simulink model "statefeedback"  (Simulink 5.0)
settings: Solver=ode1  StartTime=0.0  StopTime=1000  RelTol=1e-3
InitFcn:
  | init_c
undefined symbols (not defined in the file): a, dzcv, fc, fp, fs, g, j, l, mi, xc, yc
settings Model: LastModifiedBy=AD  BooleanDataType=off

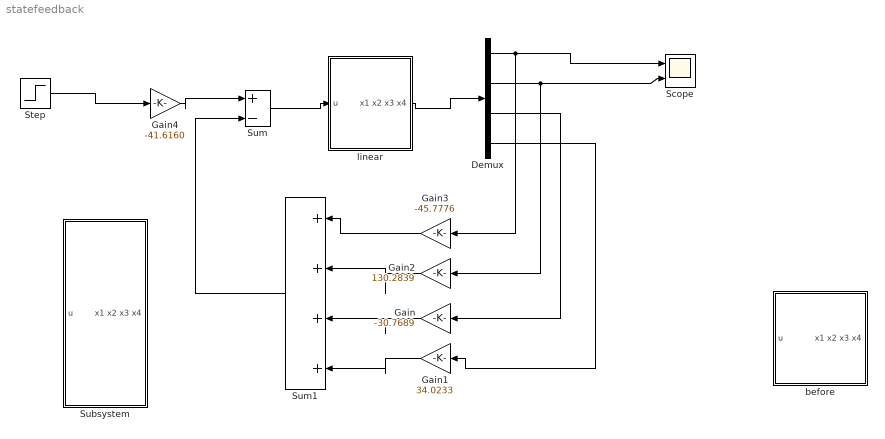
== system statefeedback ==
  Demux : Demux
  Gain : Gain  Orientation=left  Gain=-30.7689  SaturateOnIntegerOverflow=on
  Gain1 : Gain  Orientation=left  Gain=34.0233  SaturateOnIntegerOverflow=on
  Gain2 : Gain  Orientation=left  Gain=130.2839  SaturateOnIntegerOverflow=on
  Gain3 : Gain  Orientation=left  Gain=-45.7776  SaturateOnIntegerOverflow=on
  Gain4 : Gain  Gain=-41.6160  SaturateOnIntegerOverflow=on
  Scope : Scope  NumInputPorts=2
      settings: TimeRange=10  YMin=-100~0  YMax=500~120
  Step : Step  SampleTime=0
  Subsystem : Subsystem
  Sum : Sum  Inputs=|+-  SaturateOnIntegerOverflow=on
  Sum1 : Sum  Orientation=left  Inputs=|++++  SaturateOnIntegerOverflow=on
  before : Subsystem
  linear : Subsystem
  wires:
  linear/1(x1 x2 x3 x4) -> Demux/1
  Demux/1 -> Gain3/1, Scope/1
  Demux/2 -> Scope/2, Gain2/1
  Demux/3 -> Gain/1
  Demux/4 -> Gain1/1
  Gain3/1 -> Sum1/1
  Gain2/1 -> Sum1/2
  Gain/1 -> Sum1/3
  Gain1/1 -> Sum1/4
  Sum1/1 -> Sum/2
  Gain4/1 -> Sum/1
  Sum/1 -> linear/1(u)
  Step/1 -> Gain4/1

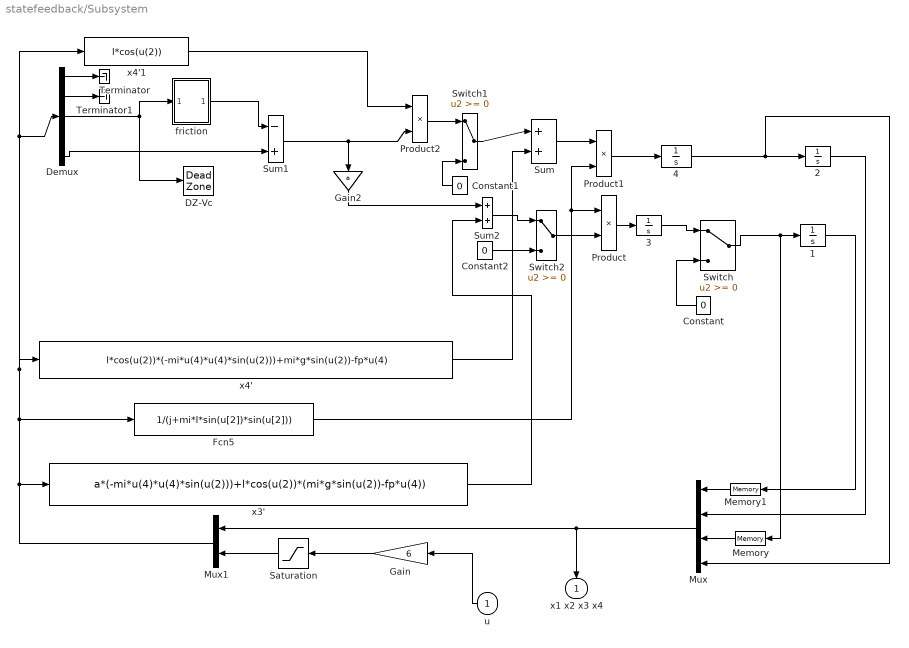
== system statefeedback/Subsystem ==
  u : Inport  Orientation=left
  {1..4} (4 alike) : Integrator
  Constant : Constant  Orientation=left  Value=0
  Constant1 : Constant  Orientation=left  Value=0
  Constant2 : Constant  Value=0
  DZ-Vc : DeadZone  LowerValue=-0.00793711  UpperValue=0.00793711  SaturateOnIntegerOverflow=on
  Demux : Demux  Outputs=5
  Fcn5 : Fcn  Expr=1/(j+mi*l*sin(u[2])*sin(u[2]))
  Gain : Gain  Orientation=left  Gain=6  SaturateOnIntegerOverflow=on
  Gain2 : Gain  Orientation=down  Gain=a  SaturateOnIntegerOverflow=on
  Memory : Memory  Orientation=left
  Memory1 : Memory  Orientation=left
  Mux : Mux  Orientation=left
  Mux1 : Mux  Orientation=left  Inputs=2
  Product : Product  SaturateOnIntegerOverflow=on
  Product1 : Product  SaturateOnIntegerOverflow=on
  Product2 : Product  SaturateOnIntegerOverflow=on
  Saturation : Saturate  Orientation=left  UpperLimit=5  LowerLimit=-5
  Sum : Sum  Inputs=|++  SaturateOnIntegerOverflow=on
  Sum1 : Sum  Inputs=-+  SaturateOnIntegerOverflow=on
  Sum2 : Sum  SaturateOnIntegerOverflow=on
  Switch : Switch  SaturateOnIntegerOverflow=on
  Switch1 : Switch  SaturateOnIntegerOverflow=on
  Switch2 : Switch  SaturateOnIntegerOverflow=on
  Terminator : Terminator
  Terminator1 : Terminator
  friction : Subsystem
  x3' : Fcn  Expr=a*(-mi*u(4)*u(4)*sin(u(2)))+l*cos(u(2))*(mi*g*sin(u(2))-fp*u(4))
  x4' : Fcn  Expr=l*cos(u(2))*(-mi*u(4)*u(4)*sin(u(2)))+mi*g*sin(u(2))-fp*u(4)
  x4'1 : Fcn  Expr=l*cos(u(2))
  x1 x2 x3 x4 : Outport  Orientation=down
  wires:
  u/1 -> Gain/1
  Demux/3 -> DZ-Vc/1, friction/1(In1)
  Constant1/1 -> Switch1/3
  Constant/1 -> Switch/3
  x4'1/1 -> Product2/1
  Product2/1 -> Switch1/1
  Switch1/1 -> Sum/1
  x4'/1 -> Sum/2
  Fcn5/1 -> Product1/2, Product/1
  Product1/1 -> 4/1
  Product/1 -> 3/1
  Gain/1 -> Saturation/1
  Mux1/1 -> x3'/1, Fcn5/1, x4'/1, x4'1/1, Demux/1
  Mux/1 -> Mux1/1, x1 x2 x3 x4/1
  Saturation/1 -> Mux1/2
  Switch/1 -> 1/1, Memory/1
  3/1 -> Switch/1
  2/1 -> Mux/2
  1/1 -> Memory1/1
  Memory/1 -> Mux/3
  Sum/1 -> Product1/1
  Switch2/1 -> Product/2
  Constant2/1 -> Switch2/3
  Memory1/1 -> Mux/1
  Sum2/1 -> Switch2/1
  x3'/1 -> Sum2/2
  Gain2/1 -> Sum2/1
  Demux/1 -> Terminator/1
  Demux/2 -> Terminator1/1
  4/1 -> 2/1, Mux/4
  Demux/5 -> Sum1/2
  Sum1/1 -> Product2/2, Gain2/1
  ? -> Switch/2, Switch1/2, Switch2/2
  friction/1(out-1) -> Sum1/1

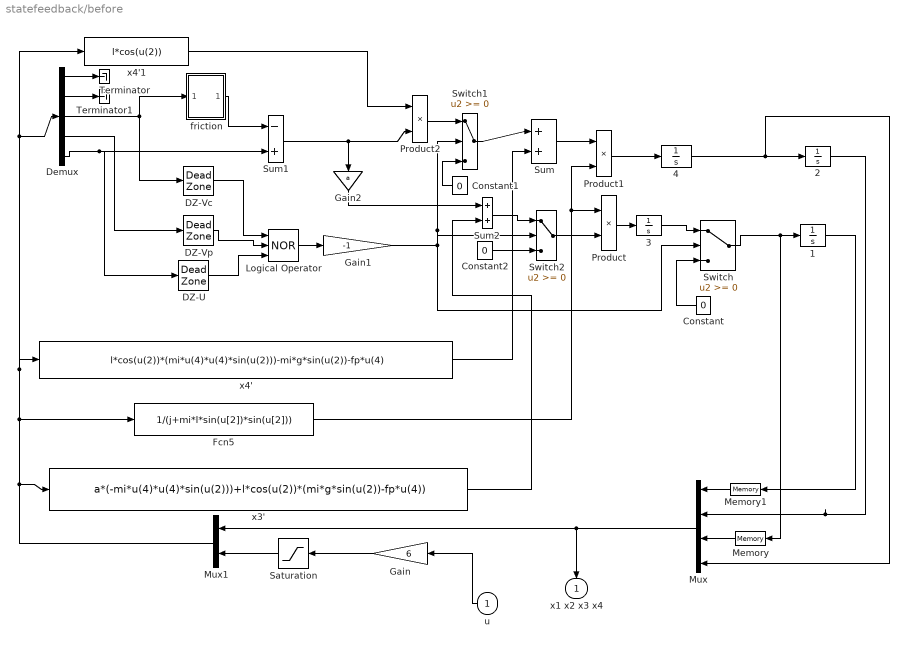
== system statefeedback/before ==
  u : Inport  Orientation=left
  {1..4} (4 alike) : Integrator
  Constant : Constant  Orientation=left  Value=0
  Constant1 : Constant  Orientation=left  Value=0
  Constant2 : Constant  Value=0
  DZ-U : DeadZone  LowerValue=-1.37918  UpperValue=1.37918  SaturateOnIntegerOverflow=on
  DZ-Vc : DeadZone  LowerValue=-0.00793711  UpperValue=0.00793711  SaturateOnIntegerOverflow=on
  DZ-Vp : DeadZone  LowerValue=-3.37476  UpperValue=3.37476  SaturateOnIntegerOverflow=on
  Demux : Demux  Outputs=5
  Fcn5 : Fcn  Expr=1/(j+mi*l*sin(u[2])*sin(u[2]))
  Gain : Gain  Orientation=left  Gain=6  SaturateOnIntegerOverflow=on
  Gain1 : Gain  Gain=-1  SaturateOnIntegerOverflow=on
  Gain2 : Gain  Orientation=down  Gain=a  SaturateOnIntegerOverflow=on
  Logical Operator : Logic  Operator=NOR  Inputs=3  AllPortsSameDT=off
  Memory : Memory  Orientation=left
  Memory1 : Memory  Orientation=left
  Mux : Mux  Orientation=left
  Mux1 : Mux  Orientation=left  Inputs=2
  Product : Product  SaturateOnIntegerOverflow=on
  Product1 : Product  SaturateOnIntegerOverflow=on
  Product2 : Product  SaturateOnIntegerOverflow=on
  Saturation : Saturate  Orientation=left  UpperLimit=5  LowerLimit=-5
  Sum : Sum  Inputs=|++  SaturateOnIntegerOverflow=on
  Sum1 : Sum  Inputs=-+  SaturateOnIntegerOverflow=on
  Sum2 : Sum  SaturateOnIntegerOverflow=on
  Switch : Switch  SaturateOnIntegerOverflow=on
  Switch1 : Switch  SaturateOnIntegerOverflow=on
  Switch2 : Switch  SaturateOnIntegerOverflow=on
  Terminator : Terminator
  Terminator1 : Terminator
  friction : Subsystem
  x3' : Fcn  Expr=a*(-mi*u(4)*u(4)*sin(u(2)))+l*cos(u(2))*(mi*g*sin(u(2))-fp*u(4))
  x4' : Fcn  Expr=l*cos(u(2))*(mi*u(4)*u(4)*sin(u(2)))-mi*g*sin(u(2))-fp*u(4)
  x4'1 : Fcn  Expr=l*cos(u(2))
  x1 x2 x3 x4 : Outport  Orientation=down
  wires:
  Gain1/1 -> Switch2/2, Switch1/2, Switch/2
  Sum1/1 -> Gain2/1, Product2/2
  Demux/5 -> Sum1/2, DZ-U/1
  4/1 -> Mux/4, 2/1
  friction/1(out-1) -> Sum1/1
  Demux/2 -> Terminator1/1
  Demux/1 -> Terminator/1
  Gain2/1 -> Sum2/1
  x3'/1 -> Sum2/2
  Sum2/1 -> Switch2/1
  Memory1/1 -> Mux/1
  Constant2/1 -> Switch2/3
  Switch2/1 -> Product/2
  Logical Operator/1 -> Gain1/1
  DZ-U/1 -> Logical Operator/3
  DZ-Vp/1 -> Logical Operator/2
  DZ-Vc/1 -> Logical Operator/1
  Sum/1 -> Product1/1
  Memory/1 -> Mux/3
  1/1 -> Memory1/1
  2/1 -> Mux/2
  3/1 -> Switch/1
  Switch/1 -> Memory/1, 1/1
  Saturation/1 -> Mux1/2
  Mux/1 -> x1 x2 x3 x4/1, Mux1/1
  Mux1/1 -> Demux/1, x4'1/1, x4'/1, Fcn5/1, x3'/1
  Gain/1 -> Saturation/1
  Product/1 -> 3/1
  Product1/1 -> 4/1
  Fcn5/1 -> Product/1, Product1/2
  x4'/1 -> Sum/2
  Switch1/1 -> Sum/1
  Product2/1 -> Switch1/1
  x4'1/1 -> Product2/1
  Constant/1 -> Switch/3
  Constant1/1 -> Switch1/3
  Demux/4 -> DZ-Vp/1
  Demux/3 -> DZ-Vc/1, friction/1(In1)
  u/1 -> Gain/1

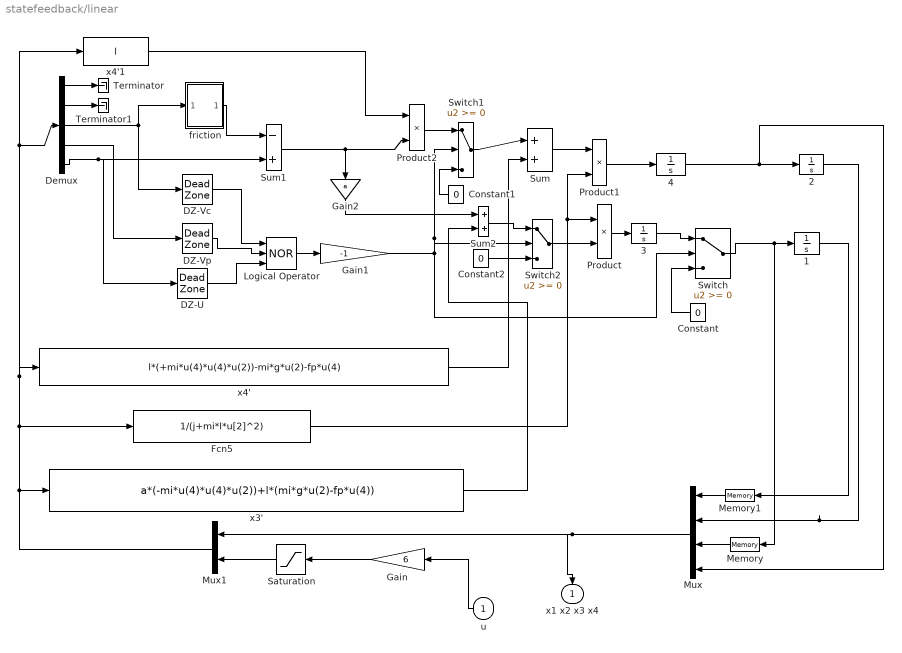
== system statefeedback/linear ==
  u : Inport  Orientation=left
  {1..4} (4 alike) : Integrator
  Constant : Constant  Orientation=left  Value=0
  Constant1 : Constant  Orientation=left  Value=0
  Constant2 : Constant  Value=0
  DZ-U : DeadZone  LowerValue=-1.37918  UpperValue=1.37918  SaturateOnIntegerOverflow=on
  DZ-Vc : DeadZone  LowerValue=-0.00793711  UpperValue=0.00793711  SaturateOnIntegerOverflow=on
  DZ-Vp : DeadZone  LowerValue=-3.37476  UpperValue=3.37476  SaturateOnIntegerOverflow=on
  Demux : Demux  Outputs=5
  Fcn5 : Fcn  Expr=1/(j+mi*l*u[2]^2)
  Gain : Gain  Orientation=left  Gain=6  SaturateOnIntegerOverflow=on
  Gain1 : Gain  Gain=-1  SaturateOnIntegerOverflow=on
  Gain2 : Gain  Orientation=down  Gain=a  SaturateOnIntegerOverflow=on
  Logical Operator : Logic  Operator=NOR  Inputs=3  AllPortsSameDT=off
  Memory : Memory  Orientation=left
  Memory1 : Memory  Orientation=left
  Mux : Mux  Orientation=left
  Mux1 : Mux  Orientation=left  Inputs=2
  Product : Product  SaturateOnIntegerOverflow=on
  Product1 : Product  SaturateOnIntegerOverflow=on
  Product2 : Product  SaturateOnIntegerOverflow=on
  Saturation : Saturate  Orientation=left  UpperLimit=5  LowerLimit=-5
  Sum : Sum  Inputs=|++  SaturateOnIntegerOverflow=on
  Sum1 : Sum  Inputs=-+  SaturateOnIntegerOverflow=on
  Sum2 : Sum  SaturateOnIntegerOverflow=on
  Switch : Switch  SaturateOnIntegerOverflow=on
  Switch1 : Switch  SaturateOnIntegerOverflow=on
  Switch2 : Switch  SaturateOnIntegerOverflow=on
  Terminator : Terminator
  Terminator1 : Terminator
  friction : Subsystem
  x3' : Fcn  Expr=a*(-mi*u(4)*u(4)*u(2))+l*(mi*g*u(2)-fp*u(4))
  x4' : Fcn  Expr=l*(+mi*u(4)*u(4)*u(2))-mi*g*u(2)-fp*u(4)
  x4'1 : Fcn  Expr=l
  x1 x2 x3 x4 : Outport  Orientation=down
  wires:
  u/1 -> Gain/1
  Demux/3 -> friction/1(In1), DZ-Vc/1
  Demux/4 -> DZ-Vp/1
  Constant1/1 -> Switch1/3
  Constant/1 -> Switch/3
  x4'1/1 -> Product2/1
  Product2/1 -> Switch1/1
  Switch1/1 -> Sum/1
  x4'/1 -> Sum/2
  Fcn5/1 -> Product1/2, Product/1
  Product1/1 -> 4/1
  Product/1 -> 3/1
  Gain/1 -> Saturation/1
  Mux1/1 -> x3'/1, Fcn5/1, x4'/1, x4'1/1, Demux/1
  Mux/1 -> Mux1/1, x1 x2 x3 x4/1
  Saturation/1 -> Mux1/2
  Switch/1 -> 1/1, Memory/1
  3/1 -> Switch/1
  2/1 -> Mux/2
  1/1 -> Memory1/1
  Memory/1 -> Mux/3
  Sum/1 -> Product1/1
  DZ-Vc/1 -> Logical Operator/1
  DZ-Vp/1 -> Logical Operator/2
  DZ-U/1 -> Logical Operator/3
  Logical Operator/1 -> Gain1/1
  Switch2/1 -> Product/2
  Constant2/1 -> Switch2/3
  Memory1/1 -> Mux/1
  Sum2/1 -> Switch2/1
  x3'/1 -> Sum2/2
  Gain2/1 -> Sum2/1
  Demux/1 -> Terminator/1
  Demux/2 -> Terminator1/1
  friction/1(out-1) -> Sum1/1
  4/1 -> 2/1, Mux/4
  Demux/5 -> DZ-U/1, Sum1/2
  Sum1/1 -> Product2/2, Gain2/1
  Gain1/1 -> Switch/2, Switch1/2, Switch2/2

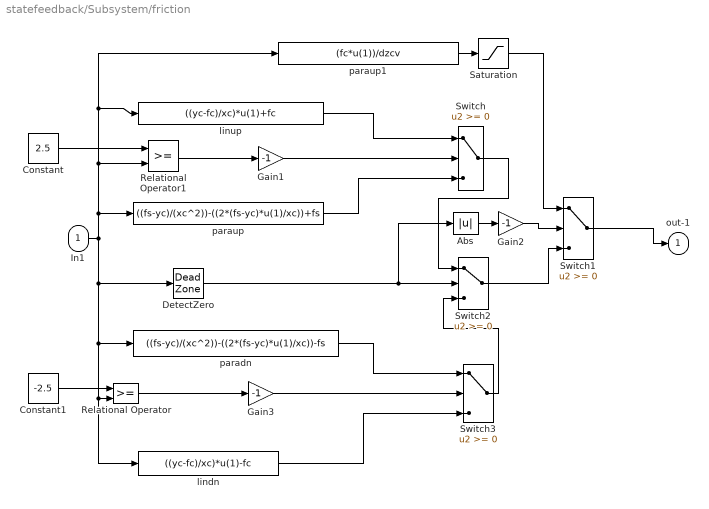
== system statefeedback/Subsystem/friction ==
  In1 : Inport
  Abs : Abs  SaturateOnIntegerOverflow=on
  Constant : Constant  Value=2.5
  Constant1 : Constant  Value=-2.5
  DetectZero : DeadZone  SaturateOnIntegerOverflow=on
  Gain1 : Gain  Gain=-1  SaturateOnIntegerOverflow=on
  Gain2 : Gain  Gain=-1  SaturateOnIntegerOverflow=on
  Gain3 : Gain  Gain=-1  SaturateOnIntegerOverflow=on
  Relational Operator : RelationalOperator
  Relational Operator1 : RelationalOperator
  Saturation : Saturate
  Switch{,1..3} (4 alike) : Switch  SaturateOnIntegerOverflow=on
  lindn : Fcn  Expr=((yc-fc)/xc)*u(1)-fc
  linup : Fcn  Expr=((yc-fc)/xc)*u(1)+fc
  paradn : Fcn  Expr=((fs-yc)/(xc^2))-((2*(fs-yc)*u(1)/xc))-fs
  paraup : Fcn  Expr=((fs-yc)/(xc^2))-((2*(fs-yc)*u(1)/xc))+fs
  paraup1 : Fcn  Expr=(fc*u(1))/dzcv
  out-1 : Outport
  wires:
  Switch1/1 -> out-1/1
  Saturation/1 -> Switch1/1
  linup/1 -> Switch/1
  paraup/1 -> Switch/3
  In1/1 -> paradn/1, Relational Operator/2, lindn/1, DetectZero/1, paraup/1, Relational Operator1/2, linup/1, paraup1/1
  DetectZero/1 -> Switch2/2, Abs/1
  Switch/1 -> Switch2/1
  Abs/1 -> Gain2/1
  Gain2/1 -> Switch1/2
  Switch2/1 -> Switch1/3
  Switch3/1 -> Switch2/3
  paradn/1 -> Switch3/1
  Relational Operator/1 -> Gain3/1
  lindn/1 -> Switch3/3
  Constant/1 -> Relational Operator1/1
  Constant1/1 -> Relational Operator/1
  Relational Operator1/1 -> Gain1/1
  paraup1/1 -> Saturation/1
  Gain1/1 -> Switch/2
  Gain3/1 -> Switch3/2

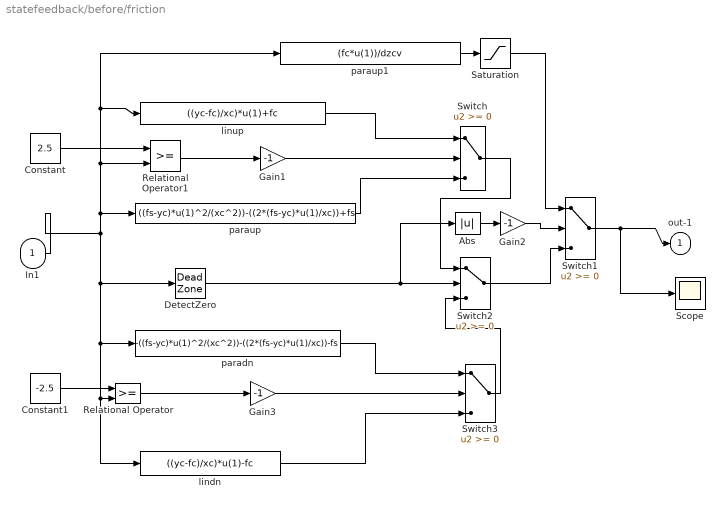
== system statefeedback/before/friction ==
  In1 : Inport
  Abs : Abs  SaturateOnIntegerOverflow=on
  Constant : Constant  Value=2.5
  Constant1 : Constant  Value=-2.5
  DetectZero : DeadZone  LowerValue=0  UpperValue=0  SaturateOnIntegerOverflow=on
  Gain1 : Gain  Gain=-1  SaturateOnIntegerOverflow=on
  Gain2 : Gain  Gain=-1  SaturateOnIntegerOverflow=on
  Gain3 : Gain  Gain=-1  SaturateOnIntegerOverflow=on
  Relational Operator : RelationalOperator
  Relational Operator1 : RelationalOperator
  Saturation : Saturate  UpperLimit=fs  LowerLimit=-fs
  Scope : Scope
      settings: SaveName=ScopeData2
  Switch{,1..3} (4 alike) : Switch  SaturateOnIntegerOverflow=on
  lindn : Fcn  Expr=((yc-fc)/xc)*u(1)-fc
  linup : Fcn  Expr=((yc-fc)/xc)*u(1)+fc
  paradn : Fcn  Expr=-((fs-yc)*u(1)^2/(xc^2))-((2*(fs-yc)*u(1)/xc))-fs
  paraup : Fcn  Expr=((fs-yc)*u(1)^2/(xc^2))-((2*(fs-yc)*u(1)/xc))+fs
  paraup1 : Fcn  Expr=(fc*u(1))/dzcv
  out-1 : Outport
  wires:
  Gain3/1 -> Switch3/2
  Gain1/1 -> Switch/2
  paraup1/1 -> Saturation/1
  Relational Operator1/1 -> Gain1/1
  Constant1/1 -> Relational Operator/1
  Constant/1 -> Relational Operator1/1
  lindn/1 -> Switch3/3
  Relational Operator/1 -> Gain3/1
  paradn/1 -> Switch3/1
  Switch3/1 -> Switch2/3
  Switch2/1 -> Switch1/3
  Gain2/1 -> Switch1/2
  Abs/1 -> Gain2/1
  Switch/1 -> Switch2/1
  DetectZero/1 -> Abs/1, Switch2/2
  paraup/1 -> Switch/3
  linup/1 -> Switch/1
  Saturation/1 -> Switch1/1
  Switch1/1 -> out-1/1, Scope/1
  In1/1 -> paraup1/1, linup/1, Relational Operator1/2, paraup/1, DetectZero/1, lindn/1, Relational Operator/2, paradn/1

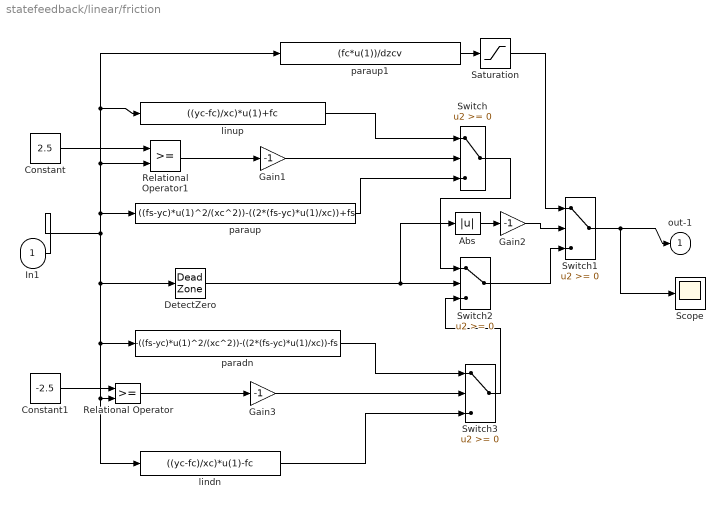
== system statefeedback/linear/friction ==
  In1 : Inport
  Abs : Abs  SaturateOnIntegerOverflow=on
  Constant : Constant  Value=2.5
  Constant1 : Constant  Value=-2.5
  DetectZero : DeadZone  LowerValue=0  UpperValue=0  SaturateOnIntegerOverflow=on
  Gain1 : Gain  Gain=-1  SaturateOnIntegerOverflow=on
  Gain2 : Gain  Gain=-1  SaturateOnIntegerOverflow=on
  Gain3 : Gain  Gain=-1  SaturateOnIntegerOverflow=on
  Relational Operator : RelationalOperator
  Relational Operator1 : RelationalOperator
  Saturation : Saturate  UpperLimit=fs  LowerLimit=-fs
  Scope : Scope
      settings: SaveName=ScopeData2
  Switch{,1..3} (4 alike) : Switch  SaturateOnIntegerOverflow=on
  lindn : Fcn  Expr=((yc-fc)/xc)*u(1)-fc
  linup : Fcn  Expr=((yc-fc)/xc)*u(1)+fc
  paradn : Fcn  Expr=-((fs-yc)*u(1)^2/(xc^2))-((2*(fs-yc)*u(1)/xc))-fs
  paraup : Fcn  Expr=((fs-yc)*u(1)^2/(xc^2))-((2*(fs-yc)*u(1)/xc))+fs
  paraup1 : Fcn  Expr=(fc*u(1))/dzcv
  out-1 : Outport
  wires:
  In1/1 -> paradn/1, Relational Operator/2, lindn/1, DetectZero/1, paraup/1, Relational Operator1/2, linup/1, paraup1/1
  Switch1/1 -> Scope/1, out-1/1
  Saturation/1 -> Switch1/1
  linup/1 -> Switch/1
  paraup/1 -> Switch/3
  DetectZero/1 -> Switch2/2, Abs/1
  Switch/1 -> Switch2/1
  Abs/1 -> Gain2/1
  Gain2/1 -> Switch1/2
  Switch2/1 -> Switch1/3
  Switch3/1 -> Switch2/3
  paradn/1 -> Switch3/1
  Relational Operator/1 -> Gain3/1
  lindn/1 -> Switch3/3
  Constant/1 -> Relational Operator1/1
  Constant1/1 -> Relational Operator/1
  Relational Operator1/1 -> Gain1/1
  paraup1/1 -> Saturation/1
  Gain1/1 -> Switch/2
  Gain3/1 -> Switch3/2
